simulink model "tutorial42_sfunction"  (R2025a)
settings: Solver=VariableStepAuto  StartTime=0.0  StopTime=10.0  RelTol=1e-3
settings Model: Creator=xing2  LastModifiedBy=xing2

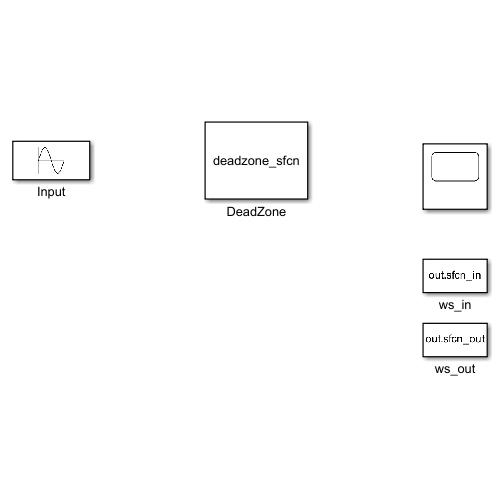
[thumbnail: Simulink's stored preview of the top-level diagram]
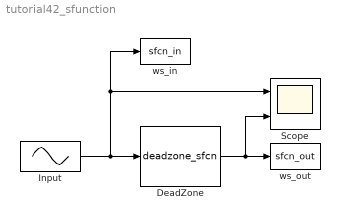
== system tutorial42_sfunction ==
  DeadZone : M-S-Function  FunctionName=deadzone_sfcn  Parameters=0.5
  Input : Sin  Amplitude=2  SampleTime=0
  Scope : Scope  NumInputPorts=2
  ws_in : ToWorkspace  VariableName=sfcn_in  SaveFormat=Timeseries  SampleTime=-1
  ws_out : ToWorkspace  VariableName=sfcn_out  SaveFormat=Timeseries  SampleTime=-1
  wires:
  Input/1 -> Scope/1, ws_in/1, DeadZone/1
  DeadZone/1 -> Scope/2, ws_out/1
